simulink model "Parawing_trim"  (R2016b)
settings: Solver=VariableStepAuto  StartTime=0.0  StopTime=200  RelTol=1e-3  EnableMultiTasking=on
PreLoadFcn:
  | parameters
values from neighbouring files (symbols this model uses):
  air_density = 1.225    [Parameters_6DOF.m]    (also in parameters.m)
  b = 7    [Parameters_6DOF.m]    (also in parameters.m)
  c = 3    [Parameters_6DOF.m]    (also in parameters.m)
  CD_0_parachute = 0.15    [Parameters_6DOF.m]    (also in parameters.m)
  CD_0_payload = 0.4    [Parameters_6DOF.m]    (also in parameters.m)
  CD_alpha_parachute = 1    [Parameters_6DOF.m]    (also in parameters.m)
  CD_alpha_payload = 2    [Parameters_6DOF.m]    (also in parameters.m)
  CD_dalpha = 0.0001    [Parameters_6DOF.m]    (also in parameters.m)
  CD_ds = 0.3    [Parameters_6DOF.m]    (also in parameters.m)
  CL_0_parachute = 0.4    [Parameters_6DOF.m]    (also in parameters.m)
  CL_alpha_parachute = 2    [Parameters_6DOF.m]    (also in parameters.m)
  CL_dalpha = 0.0001    [Parameters_6DOF.m]    (also in parameters.m)
  Cl_dalpha = 0.0021    [Parameters_6DOF.m]    (also in parameters.m)
  CL_ds = 0.21    [Parameters_6DOF.m]    (also in parameters.m)
  Cl_p = -0.1    [Parameters_6DOF.m]    (also in parameters.m)
  Cl_phi = -0.05    [parameters.m]
  Cm_0 = 0.018    [Parameters_6DOF.m]    (also in parameters.m)
  Cm_alpha = -0.2    [Parameters_6DOF.m]    (also in parameters.m)
  Cm_q = -2    [Parameters_6DOF.m]    (also in parameters.m)
  Cn_dalpha = 0.004    [Parameters_6DOF.m]    (also in parameters.m)
  Cn_r = -0.07    [Parameters_6DOF.m]    (also in parameters.m)
  gravity = 9.81    [Parameters_6DOF.m]    (also in parameters.m)
  inertia_tensor = [2.5  0   0 ... (first row only)    [Parameters_6DOF.m]    (also in parameters.m)
  inertia_tensor_inv = inertia_tensor\eye(3)    [Parameters_6DOF.m]    (also in parameters.m)
  initial_position = [0 0 -1000]'    [Main.m]    (also in parameters.m)
  initial_velocity = [13 0 0.1]'    [parameters.m]
  mass = mass_parachute + mass_body    (= 148)    [Parameters_6DOF.m]    (also in parameters.m)
  mass_matrix = diag([mass mass mass])    [Parameters_6DOF.m]    (also in parameters.m)
  mass_matrix_inv = mass_matrix\eye(3)    [Parameters_6DOF.m]    (also in parameters.m)
  S_parachute = 21    [Parameters_6DOF.m]    (also in parameters.m)
  S_payload = 0.5    [Parameters_6DOF.m]    (also in parameters.m)
undefined symbols (not defined in the file or in its folder): magnitude
libraries: aerolibutil x2, aerolibconvert2 x2, aerolibasang x1, realtime_pacer_lib x1, aerolibanim x1
settings Model: Creator=Mattia  LastModifiedBy=extra
settings DataIOCC: ExternalInput=getinputstruct(op_trim2)  InitialState=getstatestruct(op_trim2)  LoadExternalInput=on  LoadInitialState=on  SaveFormat=Array
settings OptimizationCC: LifeSpan=inf
settings DebuggingCC: SFUnexpectedBacktrackingDiag=warning  SFNoUnconditionalDefaultTransitionDiag=warning  SFExecutionAtInitializationDiag=none
settings GRTTargetCC: TargetLangStandard=C89/C90 (ANSI)  GeneratePreprocessorConditionals=Disable all
settings ConfigComp: CovMetricSettings=dw  CovHtmlReporting=on  CovSaveCumulativeToWorkspaceVar=on  CovSaveSingleToWorkspaceVar=on  CovExternalEMLEnable=off

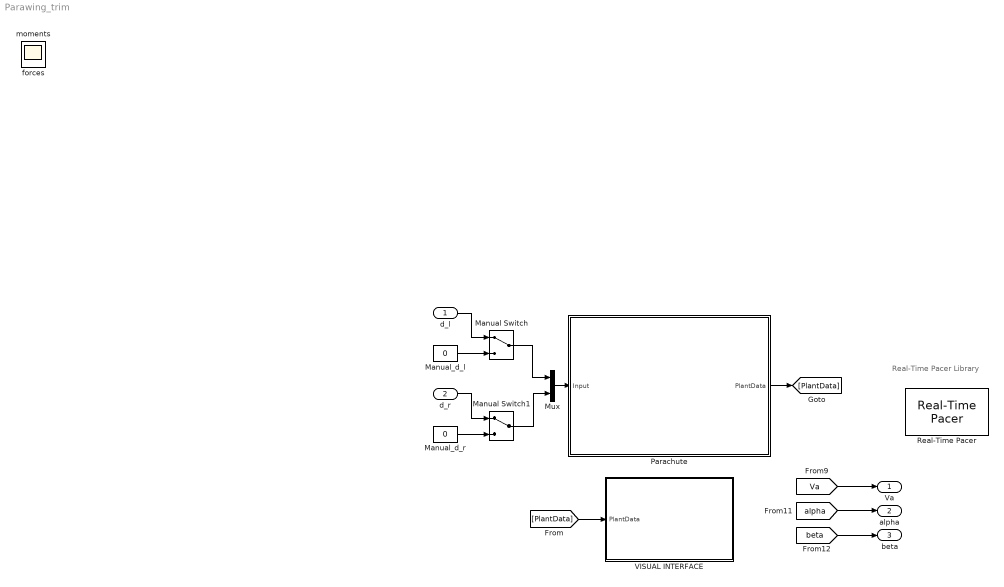
== system Parawing_trim ==
  note: Real-Time Pacer Library
  d_l : Inport
  d_r : Inport  Port=2
  Manual Switch : ManualSwitch
  Manual Switch1 : ManualSwitch
  Manual_d_l : Constant  Value=0
  Manual_d_r : Constant  Value=0
  Mux : Mux  Inputs=2
  Parachute : Subsystem
      mask Display: image('rogallo.jpg')
  Real-Time Pacer : realtime_pacer_lib/Real-Time Pacer  simTimePerRealTime=inf
  VISUAL INTERFACE : Subsystem
      mask Display: image('images/control_tower.jpg')
  Va : Outport
  alpha : Outport  Port=2
  beta : Outport  Port=3
  forces : Scope
  moments : Scope
  wires:
  Mux/1 -> Parachute/1(Input)
  Manual Switch/1 -> Mux/1
  Manual_d_l/1 -> Manual Switch/2
  Manual Switch1/1 -> Mux/2
  d_r/1 -> Manual Switch1/1
  Manual_d_r/1 -> Manual Switch1/2
  d_l/1 -> Manual Switch/1
  Parachute/1(PlantData) -> [PlantData]
  [PlantData] -> VISUAL INTERFACE/1(PlantData)
  [Va] -> Va/1
  [alpha] -> alpha/1
  [beta] -> beta/1

== system Parawing_trim/Parachute ==
  Input : Inport
  Forces and moments : Subsystem
  Vechicle Airframe Model : Subsystem
  PlantData : Outport
  wires:
  Input/1 -> Forces and moments/1(ControlInputs)
  Forces and moments/1(Forces) -> Vechicle Airframe Model/1(Forces)
  Forces and moments/2(Moments) -> Vechicle Airframe Model/2(Moments)
  Vechicle Airframe Model/1(PlantData) -> PlantData/1

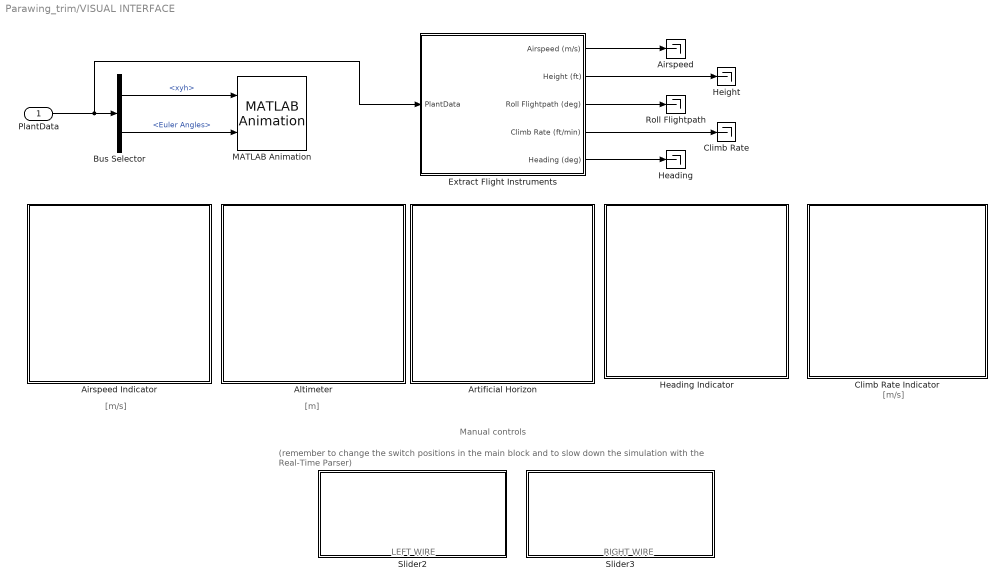
== system Parawing_trim/VISUAL INTERFACE ==
  note: (remember to change the switch positions in the main block and to slow down the simulation with the Real-Time Parser)
  note: Manual controls
  note: RIGHT WIRE
  note: LEFT WIRE
  note: [m/s]
  note: [m]
  note: [m/s]
  PlantData : Inport
  Airspeed : Terminator
  Airspeed Indicator : Subsystem  DialogController=aeroblksHMICreateDDGDialog  IsWebBlock=on  mask(MWDashboardBlock){webBlockId=1660c180-4922-4edc-b12a-b6c4fb3472e7, webBlockType=airspeedindicator, ShowInLibBrowser=on, ShowInitialText=on, HMISrcModelName=Parawing_trim}
      mask prompts: webBlockId "WebBlock Id"; webBlockType "WebBlock Type"; HMISrcModelName "Source Model"
      mask help: aeroblksHMI:aeroblkhmi:AirspeedIndicatorDialogDesc
      mask Help: eval('asbhmihelp(''airspeedindicator'')');
      mask Display:
      | if strcmp(get_param(bdroot(gcb),'BlockDiagramType'), 'library')
      |  image([(matlabroot) '/toolbox/aeroblks/aeroblks/hmi/icons/AirspeedIndicatorIcon.svg'])
      | end
  Altimeter : Subsystem  DialogController=aeroblksHMICreateDDGDialog  IsWebBlock=on  mask(MWDashboardBlock){webBlockId=dac4b64b-8b08-4b88-951c-85bcef5f9a8d, webBlockType=altimeter, ShowInLibBrowser=on, ShowInitialText=on, HMISrcModelName=Parawing_trim}
      mask prompts: webBlockId "WebBlock Id"; webBlockType "WebBlock Type"; HMISrcModelName "Source Model"
      mask help: aeroblksHMI:aeroblkhmi:AltimeterDialogDesc
      mask Help: eval('asbhmihelp(''altimeter'')');
      mask Display:
      | if strcmp(get_param(bdroot(gcb),'BlockDiagramType'), 'library')
      |  image([(matlabroot) '/toolbox/aeroblks/aeroblks/hmi/icons/AltimeterIcon.svg'])
      | end
  Artificial Horizon : Subsystem  DialogController=aeroblksHMICreateDDGDialog  IsWebBlock=on  mask(MWDashboardBlock){webBlockId=71b89583-386f-4e5a-a87e-fbc6faf0c9b0, webBlockType=artificialhorizon, ShowInLibBrowser=on, ShowInitialText=on, HMISrcModelName=Parawing_trim}
      mask prompts: webBlockId "WebBlock Id"; webBlockType "WebBlock Type"; HMISrcModelName "Source Model"
      mask help: aeroblksHMI:aeroblkhmi:ArtificialHorizonDialogDesc
      mask Help: eval('asbhmihelp(''artificialhorizon'')');
      mask Display:
      | if strcmp(get_param(bdroot(gcb),'BlockDiagramType'), 'library')
      |  image([(matlabroot) '/toolbox/aeroblks/aeroblks/hmi/icons/ArtificialHorizonIcon.svg'])
      | end
  Bus Selector : BusSelector  OutputSignals=xyh,Euler Angles
  Climb Rate : Terminator
  Climb Rate Indicator : Subsystem  DialogController=aeroblksHMICreateDDGDialog  IsWebBlock=on  mask(MWDashboardBlock){webBlockId=2290786a-142e-4cdc-9e89-cbe88d1b2ef4, webBlockType=climbindicator, ShowInLibBrowser=on, ShowInitialText=on, HMISrcModelName=Parawing_trim}
      mask prompts: webBlockId "WebBlock Id"; webBlockType "WebBlock Type"; HMISrcModelName "Source Model"
      mask help: aeroblksHMI:aeroblkhmi:ClimbIndicatorDialogDesc
      mask Help: eval('asbhmihelp(''climbindicator'')');
      mask Display:
      | if strcmp(get_param(bdroot(gcb),'BlockDiagramType'), 'library')
      |  image([(matlabroot) '/toolbox/aeroblks/aeroblks/hmi/icons/ClimbIndicatorIcon.svg'])
      | end
  Extract Flight Instruments : Subsystem
  Heading : Terminator
  Heading Indicator : Subsystem  DialogController=aeroblksHMICreateDDGDialog  IsWebBlock=on  mask(MWDashboardBlock){webBlockId=f0aafb45-9505-4aed-89ac-b6a93bae7c37, webBlockType=headingindicator, ShowInLibBrowser=on, ShowInitialText=on, HMISrcModelName=Parawing_trim}
      mask prompts: webBlockId "WebBlock Id"; webBlockType "WebBlock Type"; HMISrcModelName "Source Model"
      mask help: aeroblksHMI:aeroblkhmi:HeadingIndicatorDialogDesc
      mask Help: eval('asbhmihelp(''headingindicator'')');
      mask Display:
      | if strcmp(get_param(bdroot(gcb),'BlockDiagramType'), 'library')
      |  image([(matlabroot) '/toolbox/aeroblks/aeroblks/hmi/icons/HeadingIndicatorIcon.svg'])
      | end
  Height : Terminator
  MATLAB Animation : aerolibanim/MATLAB Animation  Tag=Matlab Animation 6 DOF  Vehicles=1  Geometries='astredwedge.mat'  BoundingBoxCoordinates=[-50,50,-50,50,-50,50]  CameraOffset=[-150,-50,0]  CameraViewAngle=5  SampleTime=0.2  FigurePosition=[1.025800e+03,4.180000e+01,1.022400e+03,1.054400e+03]
  Roll Flightpath : Terminator
  Slider2 : Subsystem  DialogController=hmiCreateDDGDialog  IsWebBlock=on  mask(MWDashboardBlock){webBlockId=dba76e04-9a7d-4e39-a6aa-4fb47b42b778, webBlockType=slider, ShowInLibBrowser=on, ShowInitialText=on, HMISrcModelName=Parawing_trim}
      mask prompts: webBlockId "WebBlock Id"; webBlockType "WebBlock Type"; HMISrcModelName "Source Model"
      mask help: SimulinkHMI:dialogs:SliderDialogDesc
      mask Help: helpview([docroot '/mapfiles/simulink.map'], 'hmi_slider')
      mask Display:
      | if strcmp(get_param(bdroot(gcb),'BlockDiagramType'), 'library')
      |     image([(matlabroot) '/toolbox/simulink/hmi/icons/Slider.png']);
      | end
  Slider3 : Subsystem  DialogController=hmiCreateDDGDialog  IsWebBlock=on  mask(MWDashboardBlock){webBlockId=f7efc1f7-4e8a-40ad-af8d-ec56bbe06b56, webBlockType=slider, ShowInLibBrowser=on, ShowInitialText=on, HMISrcModelName=Parawing_trim}
      mask prompts: webBlockId "WebBlock Id"; webBlockType "WebBlock Type"; HMISrcModelName "Source Model"
      mask help: SimulinkHMI:dialogs:SliderDialogDesc
      mask Help: helpview([docroot '/mapfiles/simulink.map'], 'hmi_slider')
      mask Display:
      | if strcmp(get_param(bdroot(gcb),'BlockDiagramType'), 'library')
      |     image([(matlabroot) '/toolbox/simulink/hmi/icons/Slider.png']);
      | end
  wires:
  Bus Selector/1 -> MATLAB Animation/1  "<xyh>"
  PlantData/1 -> Extract Flight Instruments/1(PlantData), Bus Selector/1
  Bus Selector/2 -> MATLAB Animation/2  "<Euler Angles>"
  Extract Flight Instruments/1(Airspeed (m/s)) -> Airspeed/1
  Extract Flight Instruments/2(Height (ft)) -> Height/1
  Extract Flight Instruments/4(Climb Rate (ft/min)) -> Climb Rate/1
  Extract Flight Instruments/5(Heading (deg)) -> Heading/1
  Extract Flight Instruments/3(Roll Flightpath (deg)) -> Roll Flightpath/1

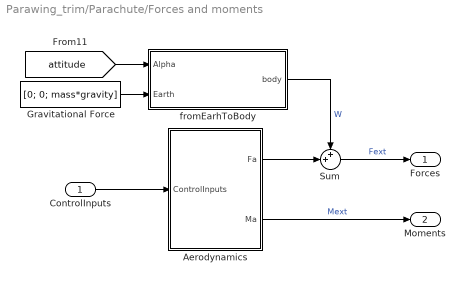
== system Parawing_trim/Parachute/Forces and moments ==
  ControlInputs : Inport
  Aerodynamics : Subsystem
  Gravitational Force : Constant  Value=[0; 0; mass*gravity]
  Sum : Sum  Inputs=++|
  fromEarhToBody : MATLAB Function  TreatAsAtomicUnit=on
  Forces : Outport
  Moments : Outport  Port=2
  wires:
  fromEarhToBody/1(body) -> Sum/1  "W"
  Sum/1 -> Forces/1  "Fext"
  [attitude] -> fromEarhToBody/1(Alpha)
  Gravitational Force/1 -> fromEarhToBody/2(Earth)
  Aerodynamics/1(Fa) -> Sum/2
  Aerodynamics/2(Ma) -> Moments/1  "Mext"
  ControlInputs/1 -> Aerodynamics/1(ControlInputs)

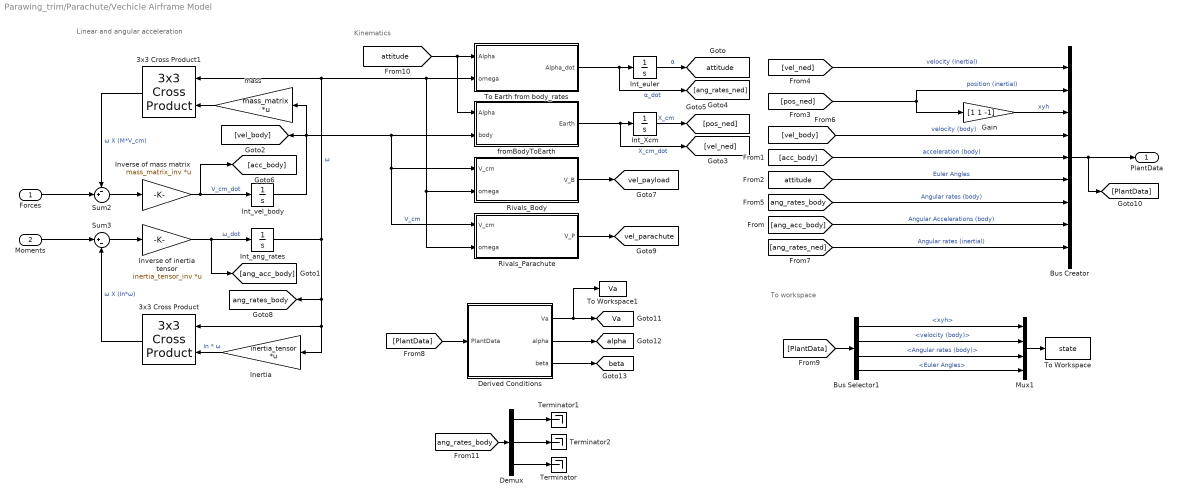
== system Parawing_trim/Parachute/Vechicle Airframe Model ==
  note: Kinematics
  note: Linear and angular acceleration
  note: To workspace
  Forces : Inport
  Moments : Inport  Port=2
  3x3 Cross Product : aerolibutil/3x3 Cross Product
  3x3 Cross Product1 : aerolibutil/3x3 Cross Product
  Bus Creator : BusCreator  Inputs='velocity (inertial)','position (inertial)','xyh','velocity (body)','acceleration (body)','Euler Angles','Angular rates (body)','Angular Accelerations (body)','Angular rates (inertial)'
  Bus Selector1 : BusSelector  OutputSignals=xyh,velocity (body),Angular rates (body),Euler Angles
  Demux : Demux  Outputs=3
  Derived Conditions : Subsystem
  Gain : Gain  Gain=[1 1 -1]
  Inertia : Gain  Gain=inertia_tensor  Multiplication=Matrix(K*u)
  Int_Xcm : Integrator  InitialCondition=initial_position
  Int_ang_rates : Integrator  InitialCondition=[0; 0; 0]
  Int_euler : Integrator  InitialCondition=[0; 0; 0]
  Int_vel_body : Integrator  InitialCondition=initial_velocity
  Inverse of inertia tensor : Gain  Gain=inertia_tensor_inv  Multiplication=Matrix(K*u)
  Inverse of mass matrix : Gain  Gain=mass_matrix_inv  Multiplication=Matrix(K*u)
  Mux1 : Mux
  Rivals_Body : MATLAB Function  TreatAsAtomicUnit=on
  Rivals_Parachute : MATLAB Function  TreatAsAtomicUnit=on
  Sum2 : Sum  Inputs=-+|
  Sum3 : Sum  Inputs=|+-
  Terminator : Terminator
  Terminator1 : Terminator
  Terminator2 : Terminator
  To Earth from body_rates : MATLAB Function  TreatAsAtomicUnit=on
  To Workspace : ToWorkspace  VariableName=state  SaveFormat=Timeseries  SampleTime=-1
      settings: Save2DSignal=2-D array (concatenate along first dimension)
  To Workspace1 : ToWorkspace  VariableName=Va  SaveFormat=Timeseries  SampleTime=-1
  fromBodyToEarth : MATLAB Function  TreatAsAtomicUnit=on
  mass : Gain  Gain=mass_matrix  Multiplication=Matrix(K*u)
  PlantData : Outport
  tag scope: Va=global, alpha=global, ang_rates_body=global, attitude=global, beta=global, vel_parachute=global, vel_payload=global
  wires:
  Forces/1 -> Sum2/2
  Moments/1 -> Sum3/1
  To Earth from body_rates/1(Alpha_dot) -> [ang_rates_ned], Int_euler/1  "α_dot"
  3x3 Cross Product/1 -> Sum3/2  "ω X (In*ω)"
  [attitude] -> fromBodyToEarth/1(Alpha), To Earth from body_rates/1(Alpha)
  Int_ang_rates/1 -> Rivals_Parachute/2(omega), Rivals_Body/2(omega), To Earth from body_rates/2(omega), 3x3 Cross Product1/1, Inertia/1, 3x3 Cross Product/1, [ang_rates_body]  "ω"
  Inverse of mass matrix/1 -> Int_vel_body/1, [acc_body]  "V_cm_dot"
  Int_vel_body/1 -> mass/1, [vel_body], Rivals_Parachute/1(V_cm), Rivals_Body/1(V_cm), fromBodyToEarth/2(body)  "V_cm"
  Sum2/1 -> Inverse of mass matrix/1
  Sum3/1 -> Inverse of inertia tensor/1
  mass/1 -> 3x3 Cross Product1/2
  Int_Xcm/1 -> [pos_ned]  "X_cm"
  Rivals_Body/1(V_B) -> [vel_payload]
  Inertia/1 -> 3x3 Cross Product/2  "In * ω"
  Int_euler/1 -> [attitude]  "α"
  Inverse of inertia tensor/1 -> [ang_acc_body], Int_ang_rates/1  "ω_dot"
  3x3 Cross Product1/1 -> Sum2/1  "ω X (M*V_cm)"
  fromBodyToEarth/1(Earth) -> [vel_ned], Int_Xcm/1  "X_cm_dot"
  Rivals_Parachute/1(V_P) -> [vel_parachute]
  [vel_ned] -> Bus Creator/1  "velocity (inertial)"
  [pos_ned] -> Bus Creator/2, Gain/1  "position (inertial)"
  Gain/1 -> Bus Creator/3  "xyh"
  [vel_body] -> Bus Creator/4  "velocity (body)"
  [acc_body] -> Bus Creator/5  "acceleration (body)"
  [attitude] -> Bus Creator/6  "Euler Angles"
  [ang_rates_body] -> Bus Creator/7  "Angular rates (body)"
  [ang_acc_body] -> Bus Creator/8  "Angular Accelerations (body)"
  [ang_rates_ned] -> Bus Creator/9  "Angular rates (inertial)"
  Bus Creator/1 -> [PlantData], PlantData/1
  Derived Conditions/2(alpha) -> [alpha]
  Derived Conditions/3(beta) -> [beta]
  Derived Conditions/1(Va) -> To Workspace1/1, [Va]
  [PlantData] -> Derived Conditions/1(PlantData)
  Bus Selector1/4 -> Mux1/4  "<Euler Angles>"
  [PlantData] -> Bus Selector1/1
  Bus Selector1/1 -> Mux1/1  "<xyh>"
  Bus Selector1/2 -> Mux1/2  "<velocity (body)>"
  Mux1/1 -> To Workspace/1
  Bus Selector1/3 -> Mux1/3  "<Angular rates (body)>"
  [ang_rates_body] -> Demux/1
  Demux/1 -> Terminator1/1
  Demux/2 -> Terminator2/1
  Demux/3 -> Terminator/1

== system Parawing_trim/VISUAL INTERFACE/Airspeed Indicator ==

== system Parawing_trim/VISUAL INTERFACE/Altimeter ==

== system Parawing_trim/VISUAL INTERFACE/Artificial Horizon ==

== system Parawing_trim/VISUAL INTERFACE/Climb Rate Indicator ==

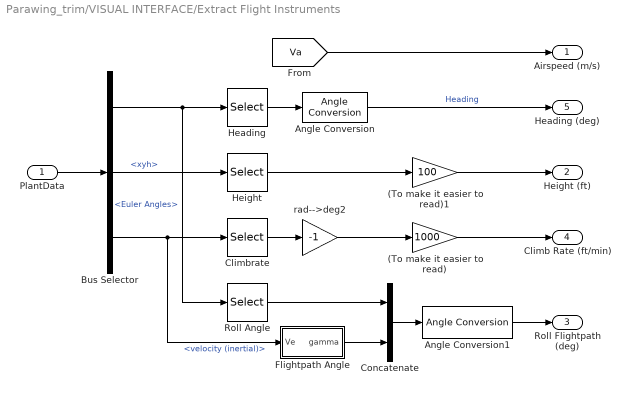
== system Parawing_trim/VISUAL INTERFACE/Extract Flight Instruments ==
  PlantData : Inport
  (To make it easier to read) : Gain  Gain=1000
  (To make it easier to read)1 : Gain  Gain=100
  Angle Conversion : aerolibconvert2/Angle Conversion  IU=rad  OU=deg
  Angle Conversion1 : aerolibconvert2/Angle Conversion  IU=rad  OU=deg
  Bus Selector : BusSelector  OutputSignals=Euler Angles,xyh,velocity (inertial)
  Climbrate : Selector  IndexMode=Zero-based  InputPortWidth=3  IndexOptions=Index vector (dialog)  Indices=2  OutputSizes=1
  Concatenate : Concatenate
  Flightpath Angle : Subsystem
  Heading : Selector  IndexMode=Zero-based  InputPortWidth=3  IndexOptions=Index vector (dialog)  Indices=2  OutputSizes=1
  Height : Selector  IndexMode=Zero-based  InputPortWidth=3  IndexOptions=Index vector (dialog)  Indices=2  OutputSizes=1
  Roll Angle : Selector  IndexMode=Zero-based  InputPortWidth=3  IndexOptions=Index vector (dialog)  Indices=0  OutputSizes=1
  rad-->deg2 : Gain  Gain=-1  SaturateOnIntegerOverflow=on  OutDataTypeStr=Inherit: Same as input  ParamDataTypeStr=Inherit: Same as input
  Airspeed (m/s) : Outport
  Height (ft) : Outport  Port=2
  Roll Flightpath (deg) : Outport  Port=3
  Climb Rate (ft/min) : Outport  Port=4
  Heading (deg) : Outport  Port=5
  wires:
  Flightpath Angle/1(gamma) -> Concatenate/2
  Angle Conversion1/1 -> Roll Flightpath (deg)/1
  Concatenate/1 -> Angle Conversion1/1
  Roll Angle/1 -> Concatenate/1
  rad-->deg2/1 -> (To make it easier to read)/1
  Bus Selector/3 -> Flightpath Angle/1(Ve), Climbrate/1  "<velocity (inertial)>"
  Climbrate/1 -> rad-->deg2/1
  Height/1 -> (To make it easier to read)1/1
  Bus Selector/2 -> Height/1  "<xyh>"
  Angle Conversion/1 -> Heading (deg)/1  "Heading"
  Heading/1 -> Angle Conversion/1
  Bus Selector/1 -> Roll Angle/1, Heading/1  "<Euler Angles>"
  [Va] -> Airspeed (m/s)/1
  PlantData/1 -> Bus Selector/1
  (To make it easier to read)/1 -> Climb Rate (ft/min)/1
  (To make it easier to read)1/1 -> Height (ft)/1

== system Parawing_trim/VISUAL INTERFACE/Heading Indicator ==

== system Parawing_trim/VISUAL INTERFACE/Slider2 ==

== system Parawing_trim/VISUAL INTERFACE/Slider3 ==

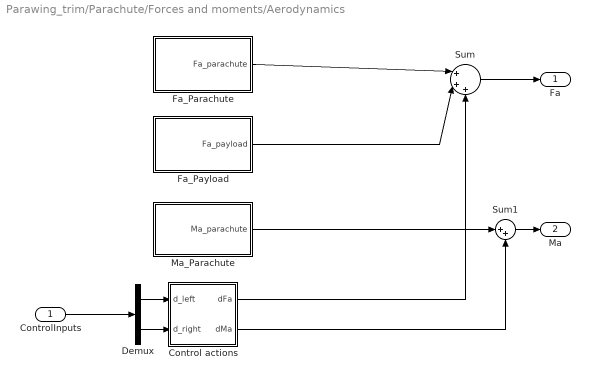
== system Parawing_trim/Parachute/Forces and moments/Aerodynamics ==
  ControlInputs : Inport
  Control actions : Subsystem
  Demux : Demux  Outputs=2
  Fa_Parachute : Subsystem
  Fa_Payload : Subsystem
  Ma_Parachute : Subsystem
  Sum : Sum  Inputs=|+++
  Sum1 : Sum  Inputs=|++
  Fa : Outport
  Ma : Outport  Port=2
  wires:
  Fa_Payload/1(Fa_payload) -> Sum/2
  Sum/1 -> Fa/1
  Fa_Parachute/1(Fa_parachute) -> Sum/1
  Sum1/1 -> Ma/1
  Demux/2 -> Control actions/2(d_right)
  ControlInputs/1 -> Demux/1
  Demux/1 -> Control actions/1(d_left)
  Control actions/1(dFa) -> Sum/3
  Ma_Parachute/1(Ma_parachute) -> Sum1/1
  Control actions/2(dMa) -> Sum1/2

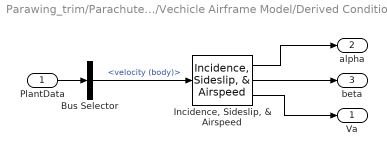
== system Parawing_trim/Parachute/Vechicle Airframe Model/Derived Conditions ==
  PlantData : Inport
  Bus Selector : BusSelector  OutputSignals=velocity (body)
  "Incidence, Sideslip, & Airspeed" : aerolibasang/Incidence, Sideslip, & Airspeed
  Va : Outport
  alpha : Outport  Port=2
  beta : Outport  Port=3
  wires:
  "Incidence, Sideslip, & Airspeed"/3 -> Va/1
  PlantData/1 -> Bus Selector/1
  "Incidence, Sideslip, & Airspeed"/1 -> alpha/1
  "Incidence, Sideslip, & Airspeed"/2 -> beta/1
  Bus Selector/1 -> "Incidence, Sideslip, & Airspeed"/1  "<velocity (body)>"

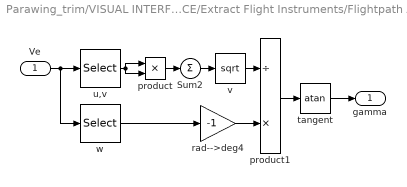
== system Parawing_trim/VISUAL INTERFACE/Extract Flight Instruments/Flightpath Angle ==
  Ve : Inport
  Sum2 : Sum  Inputs=+  SaturateOnIntegerOverflow=on  InputSameDT=on  OutDataTypeStr=Inherit: Same as first input
  product : Product  SaturateOnIntegerOverflow=on  InputSameDT=on  OutDataTypeStr=Inherit: Same as first input
  product1 : Product  Inputs=/*  SaturateOnIntegerOverflow=on  InputSameDT=on  OutDataTypeStr=Inherit: Same as first input
  rad-->deg4 : Gain  Gain=-1  SaturateOnIntegerOverflow=on  OutDataTypeStr=Inherit: Same as input  ParamDataTypeStr=Inherit: Same as input
  tangent : Trigonometry  Operator=atan
  u,v : Selector  IndexMode=Zero-based  InputPortWidth=3  IndexOptions=Index vector (dialog)  Indices=[0 1]  OutputSizes=1
  v : Sqrt  SaturateOnIntegerOverflow=on
  w : Selector  IndexMode=Zero-based  InputPortWidth=3  IndexOptions=Index vector (dialog)  Indices=2  OutputSizes=1
  gamma : Outport
  wires:
  tangent/1 -> gamma/1
  Ve/1 -> w/1, u,v/1
  product/1 -> Sum2/1
  Sum2/1 -> v/1
  product1/1 -> tangent/1
  rad-->deg4/1 -> product1/2
  v/1 -> product1/1
  u,v/1 -> product/2, product/1
  w/1 -> rad-->deg4/1

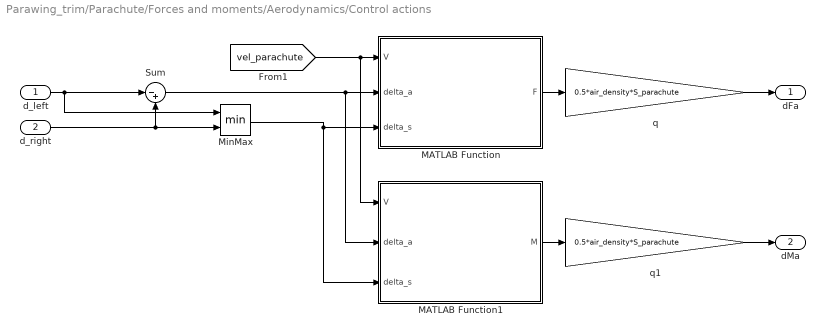
== system Parawing_trim/Parachute/Forces and moments/Aerodynamics/Control actions ==
  d_left : Inport
  d_right : Inport  Port=2
  MATLAB Function : MATLAB Function  TreatAsAtomicUnit=on
  MATLAB Function1 : MATLAB Function  TreatAsAtomicUnit=on
  MinMax : MinMax  Inputs=2
  Sum : Sum  Inputs=|-+
  q : Gain  Gain=0.5*air_density*S_parachute
  q1 : Gain  Gain=0.5*air_density*S_parachute
  dFa : Outport
  dMa : Outport  Port=2
  wires:
  MATLAB Function/1(F) -> q/1
  [vel_parachute] -> MATLAB Function1/1(V), MATLAB Function/1(V)
  q/1 -> dFa/1
  MATLAB Function1/1(M) -> q1/1
  q1/1 -> dMa/1
  d_right/1 -> Sum/2, MinMax/2
  d_left/1 -> MinMax/1, Sum/1
  Sum/1 -> MATLAB Function/2(delta_a), MATLAB Function1/2(delta_a)
  MinMax/1 -> MATLAB Function1/3(delta_s), MATLAB Function/3(delta_s)

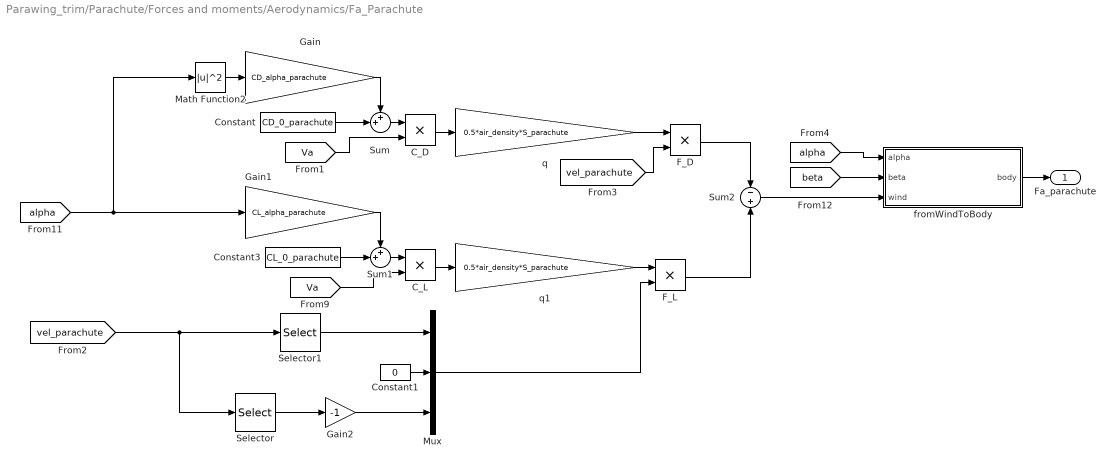
== system Parawing_trim/Parachute/Forces and moments/Aerodynamics/Fa_Parachute ==
  C_D : Product
  C_L : Product
  Constant : Constant  Value=CD_0_parachute
  Constant1 : Constant  Value=0
  Constant3 : Constant  Value=CL_0_parachute
  F_D : Product
  F_L : Product
  Gain : Gain  Gain=CD_alpha_parachute
  Gain1 : Gain  Gain=CL_alpha_parachute
  Gain2 : Gain  Gain=-1
  Math Function2 : Math  Operator=magnitude^2  SaturateOnIntegerOverflow=on
  Mux : Mux  Inputs=3
  Selector : Selector  InputPortWidth=3  IndexOptions=Index vector (dialog)  Indices=1  OutputSizes=1
  Selector1 : Selector  InputPortWidth=3  IndexOptions=Index vector (dialog)  Indices=3  OutputSizes=1
  Sum : Sum  Inputs=++|
  Sum1 : Sum  Inputs=++|
  Sum2 : Sum  Inputs=-+
  fromWindToBody : MATLAB Function  TreatAsAtomicUnit=on
  q : Gain  Gain=0.5*air_density*S_parachute
  q1 : Gain  Gain=0.5*air_density*S_parachute
  Fa_parachute : Outport
  wires:
  Math Function2/1 -> Gain/1
  Constant/1 -> Sum/2
  Gain/1 -> Sum/1
  Sum/1 -> C_D/1
  C_D/1 -> q/1
  [alpha] -> Math Function2/1, Gain1/1
  Constant3/1 -> Sum1/2
  Gain1/1 -> Sum1/1
  Sum1/1 -> C_L/1
  C_L/1 -> q1/1
  fromWindToBody/1(body) -> Fa_parachute/1
  [beta] -> fromWindToBody/2(beta)
  [Va] -> C_L/2
  q/1 -> F_D/1
  q1/1 -> F_L/1
  Selector/1 -> Gain2/1
  Gain2/1 -> Mux/3
  Selector1/1 -> Mux/1
  Constant1/1 -> Mux/2
  Mux/1 -> F_L/2
  [vel_parachute] -> F_D/2
  F_D/1 -> Sum2/1
  F_L/1 -> Sum2/2
  Sum2/1 -> fromWindToBody/3(wind)
  [vel_parachute] -> Selector/1, Selector1/1
  [Va] -> C_D/2
  [alpha] -> fromWindToBody/1(alpha)

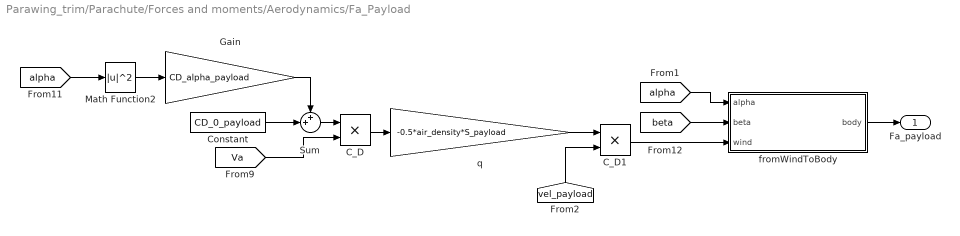
== system Parawing_trim/Parachute/Forces and moments/Aerodynamics/Fa_Payload ==
  C_D : Product
  C_D1 : Product
  Constant : Constant  Value=CD_0_payload
  Gain : Gain  Gain=CD_alpha_payload
  Math Function2 : Math  Operator=magnitude^2  SaturateOnIntegerOverflow=on
  Sum : Sum  Inputs=++|
  fromWindToBody : MATLAB Function  TreatAsAtomicUnit=on
  q : Gain  Gain=-0.5*air_density*S_payload
  Fa_payload : Outport
  wires:
  Math Function2/1 -> Gain/1
  Constant/1 -> Sum/2
  Gain/1 -> Sum/1
  Sum/1 -> C_D/1
  fromWindToBody/1(body) -> Fa_payload/1
  C_D/1 -> q/1
  [alpha] -> Math Function2/1
  [beta] -> fromWindToBody/2(beta)
  [Va] -> C_D/2
  q/1 -> C_D1/1
  C_D1/1 -> fromWindToBody/3(wind)
  [vel_payload] -> C_D1/2
  [alpha] -> fromWindToBody/1(alpha)

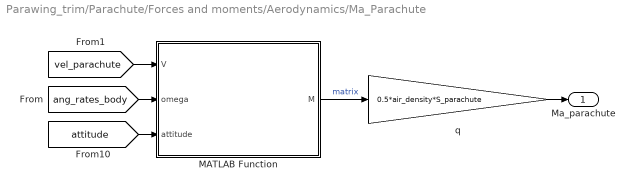
== system Parawing_trim/Parachute/Forces and moments/Aerodynamics/Ma_Parachute ==
  MATLAB Function : MATLAB Function  TreatAsAtomicUnit=on
  q : Gain  Gain=0.5*air_density*S_parachute
  Ma_parachute : Outport
  wires:
  q/1 -> Ma_parachute/1
  MATLAB Function/1(M) -> q/1  "matrix"
  [vel_parachute] -> MATLAB Function/1(V)
  [ang_rates_body] -> MATLAB Function/2(omega)
  [attitude] -> MATLAB Function/3(attitude)

== matlab function Parawing_trim/Parachute/Forces and moments/fromEarhToBody ==
  data: Alpha input; body output; Earth input
 function body = fromEarhToBody(Alpha, Earth)
%#codegen
phi = Alpha(1);
theta = Alpha(2);
psi = Alpha(3);

rotationMatrix = getEarthToBodyMatrix( phi, theta, psi );

body = rotationMatrix * Earth;

== matlab function Parawing_trim/Parachute/Vechicle Airframe Model/fromBodyToEarth ==
  data: Alpha input; Earth output; body input
 function Earth = fromBodyToEarth(Alpha, body)
%#codegen
phi = Alpha(1);
theta = Alpha(2);
psi = Alpha(3);

rotationMatrix = getEarthToBodyMatrix( phi, theta, psi )';

Earth = rotationMatrix * body;

== matlab function Parawing_trim/Parachute/Vechicle Airframe Model/To Earth from body_rates ==
  data: Alpha input; omega input; Alpha_dot output
 function Alpha_dot = Einv(Alpha, omega)
%#codegen
phi = Alpha(1);
theta = Alpha(2);

Sphi = sin(phi);
Cphi = cos(phi);
Ctheta = cos(theta);
Ttheta = tan(theta);

Einv = [1   Sphi*Ttheta    Cphi*Ttheta ;
        0       Cphi          -Sphi    ;
        0   Sphi/Ctheta    Cphi/Ctheta];

Alpha_dot = Einv * omega;

== matlab function Parawing_trim/Parachute/Vechicle Airframe Model/Rivals_Body ==
  data: V_cm input; V_B output; omega input; X_gb parameter
 function V_B = Rivals(V_cm, omega, X_gb)
%#codegen
Omega_cross = getSkew( omega );

V_B = V_cm + Omega_cross * X_gb;

== matlab function Parawing_trim/Parachute/Vechicle Airframe Model/Rivals_Parachute ==
  data: V_cm input; V_P output; omega input; X_gp parameter
 function V_P = Rivals(V_cm, omega, X_gp)
%#codegen
Omega_cross = getSkew( omega );

V_P = V_cm + Omega_cross * X_gp;

== matlab function Parawing_trim/Parachute/Forces and moments/Aerodynamics/Ma_Parachute/MATLAB Function ==
  data: V input; M output; omega input; attitude input; Cl_p parameter; Cm_q parameter; Cn_r parameter; Cl_phi parameter; Cm_0 parameter; Cm_alpha parameter; b parameter; c parameter
function M = Aero_moments(V, omega, attitude, Cl_p, Cm_q, Cn_r, Cl_phi, Cm_0, Cm_alpha, b, c)
alpha_p = atan2(V(3), V(1));
V_abs = sqrt(V(1)^2 + V(2)^2 + V(3)^2);

M = V_abs^2 * [ Cl_p * b^2 * omega(1) / (2 * V_abs ) +            Cl_phi * b * attitude(1) ;
                Cm_q * c^2 * omega(2) / (2 * V_abs ) + Cm_0 * c + Cm_alpha * c * alpha_p   ;
                Cn_r * b^2 * omega(3) / (2 * V_abs )                                      ];

== matlab function Parawing_trim/Parachute/Forces and moments/Aerodynamics/Control actions/MATLAB Function ==
  data: V input; F output; delta_a input; delta_s input; CL_dalpha parameter; CD_dalpha parameter; CL_ds parameter; CD_ds parameter
function F = Control_Forces(V, delta_a, delta_s, CL_dalpha, CD_dalpha , CL_ds, CD_ds)
V_abs = sqrt(V(1)^2 + V(2)^2 + V(3)^2);

S_F = V_abs * [ ( CL_dalpha * V(3) - CD_dalpha * V(1)) * sign(delta_a), ( CL_ds * V(3) - CD_ds * V(1))  ;
                                   - CD_dalpha * V(2)  * sign(delta_a),                - CD_ds * V(2)   ;
                (-CL_dalpha * V(1) - CD_dalpha * V(3)) * sign(delta_a), (-CL_ds * V(1) - CD_ds * V(3)) ];

F = S_F * [ delta_a  ;
            delta_s ];

== matlab function Parawing_trim/Parachute/Forces and moments/Aerodynamics/Control actions/MATLAB Function1 ==
  data: V input; M output; delta_a input; delta_s input; Cl_dalpha parameter; Cn_dalpha parameter; b parameter; t parameter
function M = Control_Moments(V, delta_a, delta_s, Cl_dalpha, Cn_dalpha, b, t)
V_abs = sqrt(V(1)^2 + V(2)^2 + V(3)^2);

S_M = V_abs^2 * [ Cl_dalpha * b / t, 0 ;
                                  0, 0 ;
                  Cn_dalpha * b / t, 0];

M = S_M * [ delta_a  ;
            delta_s ];

== matlab function Parawing_trim/Parachute/Forces and moments/Aerodynamics/Fa_Parachute/fromWindToBody ==
  data: alpha input; beta input; body output; wind input
function body = fromWindToBody(alpha, beta, wind)
%#codegen

rotationMatrix = getWindToBodyMatrix( alpha, beta );

body = rotationMatrix * wind;

== matlab function Parawing_trim/Parachute/Forces and moments/Aerodynamics/Fa_Payload/fromWindToBody ==
  data: alpha input; beta input; body output; wind input
function body = fromWindToBody(alpha, beta, wind)
%#codegen

rotationMatrix = getWindToBodyMatrix( alpha, beta );

body = rotationMatrix * wind;
